simulink model "ode45"  (R2014b)
settings: Solver=ode45  StartTime=0.0  StopTime=0.0005  FixedStep=1e-6  MaxStep=1e-4  RelTol=1e-6
values from neighbouring files (symbols this model uses):
  C = 0.04    [ode.m]
  h = 0.015    [ode.m]
  K = 0.5*10^(-4)    (= 5e-05)    [ode.m]
  L0 = 0.4*10^(-6)    (= 4e-07)    [ode.m]
  L1 = 0.4*10^(-6)    (= 4e-07)    [ode.m]
  m = 0.0012    [ode.m]
  mu = 4*pi*10^(-7)    (= 1.25663706144e-06)    [ode.m]
  R0 = 0.001    [ode.m]
  ro = 1.7*10^(-8)    (= 1.7e-08)    [ode.m]
  Ud = 100    [ode.m]
libraries: simulink x3
settings Model: Creator=marree  LastModifiedBy=marree
settings SolverCC: ConsecutiveZCsStepRelTol=1e-6  MaxConsecutiveMinStep=1000  SolverResetMethod=Robust

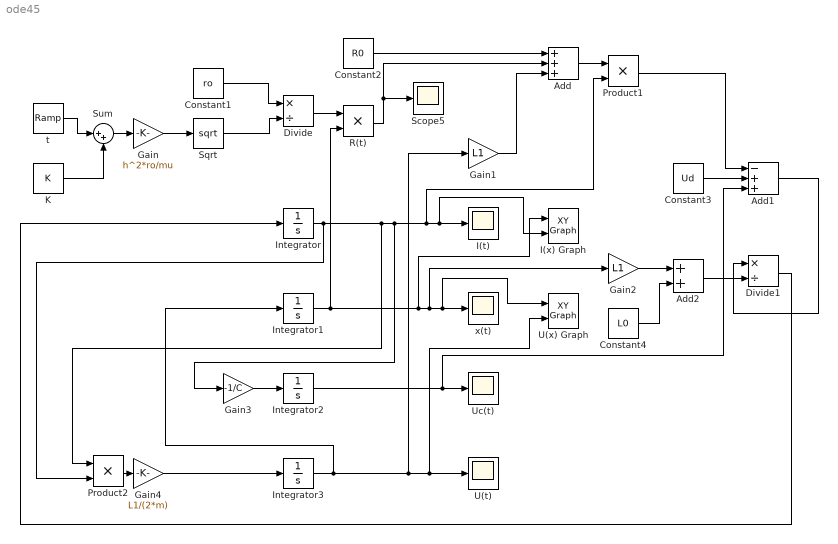
== system ode45 ==
  Add : Sum  Inputs=+++
  Add1 : Sum  Inputs=-++
  Add2 : Sum
  Constant1 : Constant  Value=ro
  Constant2 : Constant  Value=R0
  Constant3 : Constant  Value=Ud
  Constant4 : Constant  Value=L0
  Divide : Product  Inputs=*/
  Divide1 : Product  Inputs=*/
  Gain : Gain  Gain=h^2*ro/mu
  Gain1 : Gain  Gain=L1
  Gain2 : Gain  Gain=L1
  Gain3 : Gain  Gain=-1/C
  Gain4 : Gain  Gain=L1/(2*m)
  I(t) : Scope
      settings: SaveName=ScopeData3
  I(x) Graph : simulink/Sinks/XY Graph  xmin=0  xmax=1  ymin=0  ymax=600000  st=-1
  Integrator : Integrator
  Integrator1 : Integrator
  Integrator2 : Integrator  InitialCondition=2000
  Integrator3 : Integrator  InitialCondition=200
  K : Constant  Value=K
  Product1 : Product
  Product2 : Product
  R(t) : Product
  Scope5 : Scope
      settings: SaveName=ScopeData5
  Sqrt : Sqrt  SaturateOnIntegerOverflow=on
  Sum : Sum  Inputs=|++
  U(t) : Scope
  U(x) Graph : simulink/Sinks/XY Graph  xmin=0  xmax=1  ymin=0  ymax=6000  st=-1
  Uc(t) : Scope
      settings: SaveName=ScopeData2
  t : simulink/Sources/Ramp  slope=1  start=0  X0=0
  x(t) : Scope
  wires:
  K/1 -> Sum/2
  t/1 -> Sum/1
  Sum/1 -> Gain/1
  Gain/1 -> Sqrt/1
  Constant1/1 -> Divide/1
  Sqrt/1 -> Divide/2
  Divide/1 -> R(t)/1
  Integrator1/1 -> I(x) Graph/1, x(t)/1, U(x) Graph/1, Gain2/1, R(t)/2
  Constant2/1 -> Add/1
  R(t)/1 -> Scope5/1, Add/2
  Gain1/1 -> Add/3
  Add/1 -> Product1/1
  Product1/1 -> Add1/1
  Constant3/1 -> Add1/2
  Integrator2/1 -> Add1/3, Uc(t)/1
  Gain2/1 -> Add2/1
  Constant4/1 -> Add2/2
  Add1/1 -> Divide1/1
  Add2/1 -> Divide1/2
  Divide1/1 -> Integrator/1
  Gain3/1 -> Integrator2/1
  Product2/1 -> Gain4/1
  Gain4/1 -> Integrator3/1
  Integrator/1 -> I(t)/1, I(x) Graph/2, Product1/2, Gain3/1, Product2/1, Product2/2
  Integrator3/1 -> U(t)/1, U(x) Graph/2, Gain1/1, Integrator1/1
